simulink model "AlgebraicDesign_UnstablePlant_sim"  (R2025b)
settings: Solver=VariableStepAuto  StartTime=0.0  StopTime=t_sim  RelTol=1e-3
values from neighbouring files (symbols this model uses):
  delta1 = 1    [AlgebraicDesign_PolePlacement.m]
  delta2 = 1    [AlgebraicDesign_PolePlacement.m]
  rho = 1    [AlgebraicDesign_PolePlacement.m]
  Ts = 5e-3    (= 0.005)    [AlgebraicDesign_PolePlacement.m]    (also in ClosedLoop_1DOF_Analysis.m = 1)
libraries: cstblocks x2, simulink x1
settings Model: Creator=nicol  LastModifiedBy=nicol

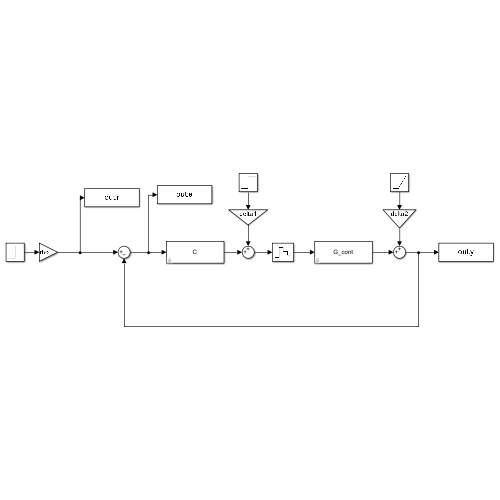
[thumbnail: Simulink's stored preview of the top-level diagram]
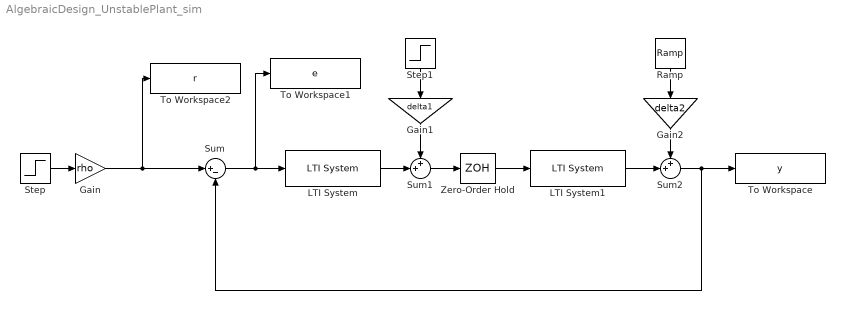
== system AlgebraicDesign_UnstablePlant_sim ==
  Gain : Gain  Gain=rho
  Gain1 : Gain  Gain=delta1
  Gain2 : Gain  Gain=delta2
  LTI System : cstblocks/LTI System  sys=C  IC=[]  PadeOrder=0
  LTI System1 : cstblocks/LTI System  sys=G_cont  IC=[]  PadeOrder=0
  Ramp : simulink/Sources/Ramp  slope=0.1  start=0  InitialOutput=0
  Step : Step  Time=0  SampleTime=0
  Step1 : Step  Time=0  After=0.7  SampleTime=0
  Sum : Sum  Inputs=|+-
  Sum1 : Sum  Inputs=++|
  Sum2 : Sum  Inputs=++|
  To Workspace : ToWorkspace  VariableName=y  SaveFormat=Structure With Time  SampleTime=-1
  To Workspace1 : ToWorkspace  VariableName=e  SaveFormat=Timeseries  SampleTime=-1
  To Workspace2 : ToWorkspace  VariableName=r  SaveFormat=Timeseries  SampleTime=-1
  Zero-Order Hold : ZeroOrderHold  SampleTime=Ts
  wires:
  Sum/1 -> LTI System/1, To Workspace1/1
  Sum2/1 -> Sum/2, To Workspace/1
  Sum1/1 -> Zero-Order Hold/1
  Step1/1 -> Gain1/1
  LTI System/1 -> Sum1/2
  LTI System1/1 -> Sum2/2
  Zero-Order Hold/1 -> LTI System1/1
  Step/1 -> Gain/1
  Ramp/1 -> Gain2/1
  Gain/1 -> To Workspace2/1, Sum/1
  Gain1/1 -> Sum1/1
  Gain2/1 -> Sum2/1
